simulink model "ClosedLoopPMSM_ASMO_MPC"  (R2023b)
settings: Solver=ode4  StartTime=0.0  StopTime=3  FixedStep=1e-6  RelTol=1e-4
InitFcn:
  | Vdc=24;
  | Rs=0.05734;
  | Ld=1.8166e-05;
  | Lq=1.8166e-05;
  | Ls=1.8166e-05;
  | pm=0.0185;
  | P=14;
  | B=1e-4;
  | J=2.94e-5;
  | Tpwm=30e-6;
  | 
  | fc=20;
  | mag_vel=100;
undefined symbols (not defined in the file): DiscIntNeverNeededParam
libraries: simulink x3, spsThreePhaseVIMeasurementLib x2, spsDCVoltageSourceLib x2, slpidlib x2, spsThreeLevelBridgeLib x1, spsUniversalBridgeLib x1, spsPermanentMagnetSynchronousMachineLib x1, sps_lib x1
(part 2 of 2)

== matlab function ClosedLoopPMSM_ASMO_MPC/ASMO/adaptive_gain ==
  data: k_alpha input; k_beta input; S_alpha input; S_beta input; H_alpha input; H_beta input; dk_alpha output; dk_beta output; dphi_alpha output; dphi_beta output; phi_alpha input; phi_beta input; K1_alpha input; K1_beta input; dK1_alpha output; dK1_beta output
function [dk_alpha, dk_beta, dphi_alpha, dphi_beta, dK1_alpha, dK1_beta] = adaptive_gain( ...
    k_alpha, k_beta, S_alpha, S_beta, H_alpha, H_beta, phi_alpha, phi_beta, K1_alpha, K1_beta)

    % Inputs:
    %   S_alpha, S_beta : Gia tri mat truot hien tai
    %   H_alpha, H_beta : Gia tri ham chuyen mach mem (tanh) hien tai
    %   k_alpha, k_beta : He so truot thich nghi k(t) cho buoc hien tai
    %   phi             : Gia tri hien tai cua phi 
    %   K1              : Gia tri luu tru cua K1 
    
    % Outputs:
    %   dk_apha, beta   : Dao ham theo thoi gian cua k_alpha, beta
    %   dphi            : Dao ham theo thoi gian cua phi (dphi/dt)
    %   dK1             : Dao ham cua bien nho K1
    
    %% Tham so
    K0      = 150;            % Toc do thich nghi
    tau     = 0.001;         % Hang so thoi gian bo loc
    epsilon = 0.5;            % Nguong xac dinh S gan 0
    gamma   = 1000;            % He so hoi tu nhanh ve gia tri K mong muon khi toi mat truot
    % GIOI HAN AN TOAN (Tranh k tang len vo cuc)
    MAX_K_DERIVATIVE = 100000; 
    MAX_K_VAL = 1500; % Neu k hien tai > 5000 thi ngung tang

    %% Tinh dao ham cua bo loc phi (Low-pass filter dynamics)
    % dphi/dt = (H - phi) / tau
    dphi_alpha = (H_alpha - phi_alpha) / tau;
    dphi_beta = (H_beta - phi_beta) / tau;

    %% Tinh dao ham cua he so k va K1 (Adaptive Law)
    if abs(S_alpha) > epsilon
        % --- Giai doan 1: Reaching Phase (|S| != 0) ---
        % dk/dt = K0 * |S|
        if k_alpha > MAX_K_VAL
            dk_alpha = 0; % Ngat tich phan neu k qua lon
        else
            dk_alpha = K0 * abs(S_alpha);
        end
        % Dat dK1/dt = dk/dt de K1 luon cap nhat bang k.
        dK1_alpha = dk_alpha;      
    else
        % --- Giai doan 2: Sliding Phase (|S| = 0) ---
        % k(t) = K1 * sqrt(|phi|)
        target_k_alpha = K1_alpha * sqrt(abs(phi_alpha));
        % dk/dt = gamma * (Target - Current)
        raw_dk_alpha = gamma * (target_k_alpha - k_alpha);
        % Bao hoa dao ham (tranh shock)
        dk_alpha = max(min(raw_dk_alpha, MAX_K_DERIVATIVE), -MAX_K_DERIVATIVE);
        % Trong giai doan nay, K1 giu nguyen gia tri
        dK1_alpha = 0;
    end

    if abs(S_beta) > epsilon
        % --- Giai doan 1: Reaching Phase (|S| != 0) ---
        % dk/dt = K0 * |S|
        if k_beta > MAX_K_VAL
            dk_beta = 0; 
        else
            dk_beta = K0 * abs(S_beta);
        end
        % Dat dK1/dt = dk/dt de K1 luon cap nhat bang k.      
        dK1_beta = dk_beta;
    else
        % --- Giai doan 2: Sliding Phase (|S| = 0) ---
        % k(t) = K1 * sqrt(|phi|)
        target_k_beta = K1_beta * sqrt(abs(phi_beta));
        % dk/dt = gamma * (Target - Current)
        raw_dk_beta = gamma * (target_k_beta - k_beta);
        % Bao hoa dao ham (tranh shock)
        dk_beta = max(min(raw_dk_beta, MAX_K_DERIVATIVE), -MAX_K_DERIVATIVE);
        % Trong giai doan nay, K1 giu nguyen gia tri
        dK1_beta = 0;
    end
end

== matlab function ClosedLoopPMSM_ASMO_MPC/SVPWM/SVPWM_main/T1T2 Calculate ==
  settings: fimath=|
      | fimath(...
      | 'RoundMode', 'floor',...
      | 'OverflowMode', 'wrap',...
      | 'ProductMode', 'KeepLSB', 'ProductWordLength', 32,...
      | 'SumMode', 'KeepLSB', 'SumWordLength', 32,...
      | 'CastBeforeSum', false)
  data: N input; T1 output; XYZ input; Tpwm input; T2 output
function [T1, T2] = T1T2_calc(N, XYZ, Tpwm)

    X = XYZ(1);
    Y = XYZ(2);
    Z = XYZ(3);

    % Default
    T1 = 0;
    T2 = 0;

    switch N
        case 1
            T1 = Z;   T2 = Y;
        case 2
            T1 = Y;   T2 = -X;
        case 3
            T1 = -Z;  T2 = X;
        case 4
            T1 = -X;  T2 = Z;
        case 5
            T1 = X;  T2 = -Y;
        case 6
            T1 = -Y;   T2 = -Z;
        otherwise
    end

    % Chuan hoa de dam bao T1 + T2 <= Tpwm
    if (T1 + T2) > Tpwm && (T1 + T2) > 0
        T1 = Tpwm * T1 / (T1 + T2);
        T2 = Tpwm * T2 / (T1 + T2);
    end
end

== matlab function ClosedLoopPMSM_ASMO_MPC/SVPWM/SVPWM_main/Tcm Calculate ==
  settings: fimath=|
      | fimath(...
      | 'RoundMode', 'floor',...
      | 'OverflowMode', 'wrap',...
      | 'ProductMode', 'KeepLSB', 'ProductWordLength', 32,...
      | 'SumMode', 'KeepLSB', 'SumWordLength', 32,...
      | 'CastBeforeSum', false)
  data: N input; Tcm1 output; T1 input; T2 input; Tcm2 output; Tpwm input; Tcm3 output
function [Tcm1, Tcm2, Tcm3] = Tcm_calc(N, T1, T2, Tpwm)
%Chuan hoa qua duty
a = (Tpwm - T1 - T2)/4; %T0/4
b = a + 0.5*T1;         %T0/4+T1/2
c = b + 0.5*T2;         %T0/4+T1/2+T2/2

% Gan theo sector
switch N
    case 1
        Tcm1 = b; Tcm2 = a; Tcm3 = c;
    case 2
        Tcm1 = a; Tcm2 = c; Tcm3 = b;
    case 3
        Tcm1 = a; Tcm2 = b; Tcm3 = c;
    case 4
        Tcm1 = c; Tcm2 = b; Tcm3 = a;
    case 5
        Tcm1 = c; Tcm2 = a; Tcm3 = b;
    case 6
        Tcm1 = b; Tcm2 = c; Tcm3 = a;
    otherwise
        Tcm1 = 0; Tcm2 = 0; Tcm3 = 0;
end

end

== matlab function ClosedLoopPMSM_ASMO_MPC/ASMO/current_observer ==
  data: S_alpha output; S_beta output; H_alpha output; H_beta output; e_err_alpha output; e_err_beta output; k_alpha input; k_beta input; di_est_alpha output; di_est_beta output; i_err_alpha output; i_err_beta output; ualpha input; ubeta input; ialpha input; ibeta input; Rs input; Ls input; e_est_alpha input; e_est_beta input; i_est_alpha input; i_est_beta input; int_e_alpha input; int_e_beta input
function [S_alpha, S_beta, H_alpha, H_beta, e_err_alpha, e_err_beta, di_est_alpha, di_est_beta, i_err_alpha, i_err_beta] = ...
    current_observer( k_alpha, k_beta, ualpha, ubeta, ialpha, ibeta, Rs, Ls, e_est_alpha, e_est_beta, i_est_alpha, i_est_beta, int_e_alpha, int_e_beta)

    % Inputs:
    %   ualpha, ubeta       : Dien ap do duoc (Stator voltage)
    %   ialpha, ibeta       : Dong dien do duoc (Measured current)
    %   Rs, Ls              : Dien tro va dien cam Stator
    %   i_est_alpha, beta   : Dong dien uoc luong (Estimated current) 
    %   int_e_alpha, beta   : Tich phan sai so dong dien (Integral of current error) 
    %   e_est_alpha, beta   : Back-EMF uoc luong (tu Back-EMF Observer 
    %   k_alpha, k_beta     : He so truot thich nghi (Adaptive gain) 
    
    % Outputs:
    %   di_est_alpha, beta  : Dao ham dong dien uoc luong 
    %   dk_alpha, beta      : Dao ham he so k 
    %   e_err_alpha, beta   : Sai so Back-EMF 
    %   S_alpha, S_beta     : Gia tri mat truot hien tai
    %   H_alpha, H_beta     : Gia tri ham chuyen mach mem (tanh) hien tai

    %% Tham so
    chi    = 15;    %giam rung, tang toc do hoi tu
    a      = 8;     %do day lop bien -> tang toc do hoi tu 

    %% Tinh toan sai so dong dien va back-EMF uoc luong
    % i_err = i_est - i_meas
    i_err_alpha = i_est_alpha - ialpha;
    i_err_beta  = i_est_beta  - ibeta;

    e_err_alpha = (chi*Ls - Rs) * i_err_alpha;
    e_err_beta = (chi*Ls - Rs) * i_err_beta;

    %% Tinh toan ham truot 
    % S = i_err + lambda * integral(i_err)
    S_alpha = i_err_alpha + chi * int_e_alpha;
    S_beta  = i_err_beta  + chi * int_e_beta;

    %% Ham chuyen mach 
    % H(S) = (e^(a*S) - e^(-a*S)) / (e^(a*S) + e^(-a*S))
    % H_alpha = (exp(a * S_alpha) - exp(-a * S_alpha)) / (exp(a * S_alpha) + exp(-a * S_alpha));
    % H_beta  = (exp(a * S_beta) - exp(-a * S_beta)) / (exp(a * S_beta) + exp(-a * S_beta));
    
    % H_alpha = tanh(a * S_alpha);
    % H_beta  = tanh(a * S_beta);
    % % H(S) = (2 / (1 + e^(-a*S))) - 1
    H_alpha = (2 / (1 + exp(-a * S_alpha))) - 1;
    H_beta  = (2 / (1 + exp(-a * S_beta))) - 1;

    %% Tinh toan dao ham dong dien uoc luong
    % di_est/dt = -Rs * i_est/Ls  + 1/Ls * (u - e_est) - k * H/Ls
    di_est_alpha = (-Rs * i_est_alpha/Ls ) + ualpha/Ls - e_est_alpha/Ls - k_alpha * H_alpha/Ls;
    di_est_beta  = (-Rs * i_est_beta/Ls )  + ubeta/Ls - e_est_beta/Ls - k_beta * H_beta/Ls;

end

== matlab function ClosedLoopPMSM_ASMO_MPC/SVPWM/SVPWM_main/Sector Calculate ==
  settings: fimath=|
      | fimath(...
      | 'RoundMode', 'floor',...
      | 'OverflowMode', 'wrap',...
      | 'ProductMode', 'KeepLSB', 'ProductWordLength', 32,...
      | 'SumMode', 'KeepLSB', 'SumWordLength', 32,...
      | 'CastBeforeSum', false)
  data: Valpha input; N output; Vbeta input
function N = sector_identification(Valpha, Vbeta)

    % DK A
    if Vbeta > 0
        A = 1;
    else
        A = 0;
    end

    % DK B
    if (sqrt(3)*Valpha - Vbeta) > 0
        B = 1;
    else
        B = 0;
    end

    %DK C
    if (-sqrt(3)*Valpha - Vbeta) > 0
        C = 1;
    else
        C = 0;
    end

    % Tinh sector
    N = A + 2*B + 4*C;
end
